simulink model "Quadrature"  (R2024b)
settings: Solver=FixedStepAuto  StartTime=0.0  StopTime=inf  FixedStep=0.1  RelTol=1e-3  EnableMultiTasking=on
libraries: stm32f4xxblockslib x5, stm32g4xxblockslib x3
settings Model: STM32="{\"EncoderBlockForG4\":[{\"ID\":\"Quadrature:1\"},{\"ID\":\"Quadrature:14\"},{\"ID\":\"Quadrature:22\"}],\"DigitalPortRead\":[{\"ID\":\"Quadrature:4\"},{\"ID\":\"Quadrature:10\"},{\"ID\":\"Quadrature:18\"},{\"ID\":\"Quadrature:26\"},{\"ID\":\"Quadrature:27\"}]}"  Creator=spwkp  LastModifiedBy=spwkp
settings OptimizationCC: DefaultParameterBehavior=Inlined  EnhancedBackFolding=on  PassReuseOutputArgsAs=Individual arguments  ZeroExternalMemoryAtStartup=off  ZeroInternalMemoryAtStartup=off  MaxStackSize=512  OptimizeBlockOrder=speed  DifferentSizesBufferReuse=on  OptimizationCustomize=off  EfficientTunableParamExpr=on
settings DebuggingCC: ParameterTunabilityLossMsg=error
settings HardwareCC: ProdBitPerPointer=32  ProdBitPerSizeT=32  ProdBitPerPtrDiffT=32  ProdLargestAtomicInteger=Long  ProdLargestAtomicFloat=Double  ProdWordSize=32  ProdLongLongMode=on  ProdHWDeviceType=ARM Compatible->ARM Cortex-M
settings SFSimCC: MATLABDynamicMemAlloc=off
settings RTWCC: Description=Embedded Coder  SystemTargetFile=ert.tlc  HardwareBoard=STM32G4xx Based  TemplateMakefile=ert_default_tmf  Toolchain=GNU Tools for ARM Embedded Processors
settings CodeAppCC: ForceParamTrailComments=on  IgnoreCustomStorageClasses=off  OperatorAnnotations=on  SimulinkDataObjDesc=on  SFDataObjDesc=on  InsertBlockDesc=on
settings ERTTargetCC: TargetLangStandard=C99 (ISO)  CodeReplacementLibrary=ARM Cortex-M  ExtModeTransport=3  ExtModeStaticAlloc=on  ExtModeStaticAllocSize=2048  ExtModeMexFile=ext_xcp  ExtModeIntrfLevel=Level2 - Open

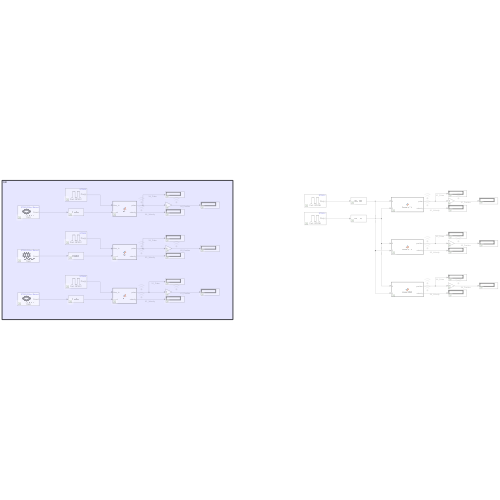
[thumbnail: Simulink's stored preview of the top-level diagram]
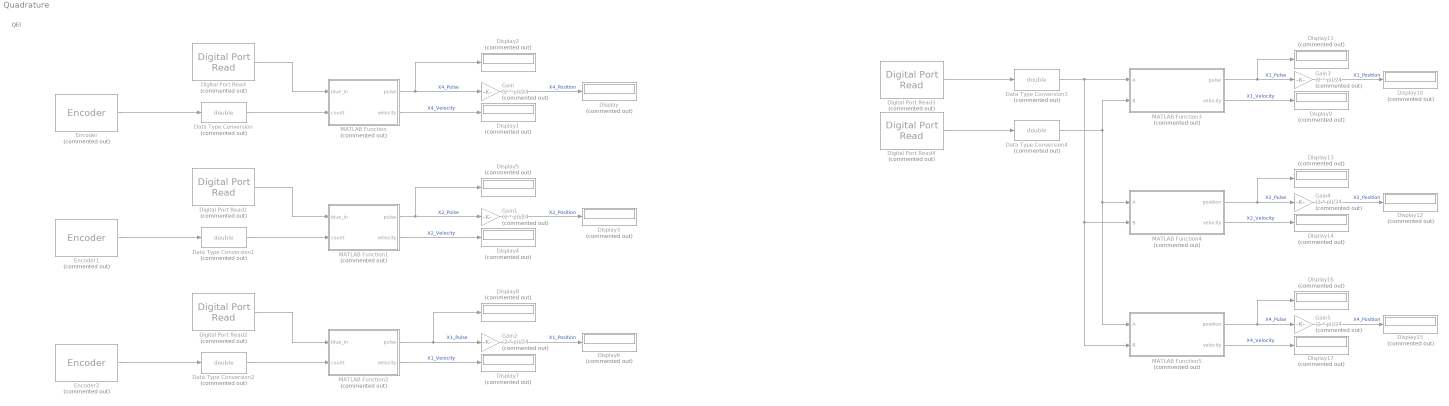
== system Quadrature ==
  note: QEI
  Data Type Conversion{,1..4} (5 alike) : DataTypeConversion  Commented=on  OutDataTypeStr=double  SaturateOnIntegerOverflow=off  RndMeth=Floor
  Digital Port Read : stm32f4xxblockslib/Digital Port Read  Commented=on  PortName=GPIOC  PinNumber=[13]  ReadOperation=on  IOAsArray=on  SampleTime=-1  EnableSimPort=off  hoistedMaskSrc=ECSoC/ECSimCodegen/Digital Port Read
      settings: LibrarySourceBlock=stm32g4xxblockslib/Digital Port Read
  Digital Port Read1 : stm32f4xxblockslib/Digital Port Read  Commented=on  PortName=GPIOC  PinNumber=[13]  ReadOperation=on  IOAsArray=on  SampleTime=-1  EnableSimPort=off  hoistedMaskSrc=ECSoC/ECSimCodegen/Digital Port Read
      settings: LibrarySourceBlock=stm32g4xxblockslib/Digital Port Read
  Digital Port Read2 : stm32f4xxblockslib/Digital Port Read  Commented=on  PortName=GPIOC  PinNumber=[13]  ReadOperation=on  IOAsArray=on  SampleTime=-1  EnableSimPort=off  hoistedMaskSrc=ECSoC/ECSimCodegen/Digital Port Read
      settings: LibrarySourceBlock=stm32g4xxblockslib/Digital Port Read
  Digital Port Read3 : stm32f4xxblockslib/Digital Port Read  Commented=on  PortName=GPIOB  PinNumber=[13]  ReadOperation=on  IOAsArray=on  SampleTime=-1  EnableSimPort=off  hoistedMaskSrc=ECSoC/ECSimCodegen/Digital Port Read
      settings: LibrarySourceBlock=stm32g4xxblockslib/Digital Port Read
  Digital Port Read4 : stm32f4xxblockslib/Digital Port Read  Commented=on  PortName=GPIOB  PinNumber=[14]  ReadOperation=on  IOAsArray=on  SampleTime=-1  EnableSimPort=off  hoistedMaskSrc=ECSoC/ECSimCodegen/Digital Port Read
      settings: LibrarySourceBlock=stm32g4xxblockslib/Digital Port Read
  Display{,1..17} (18 alike) : Display  Commented=on
  Encoder : stm32g4xxblockslib/Encoder  Commented=on  TimerModule=TIM3  EnableResetInput=off  OutputCountAfterFirstIndex=off  OutputValidIndex=off  OutputDirection=off  OutputStatus=off  SampleTime=-1
  Encoder1 : stm32g4xxblockslib/Encoder  Commented=on  TimerModule=TIM4  EnableResetInput=off  OutputCountAfterFirstIndex=off  OutputValidIndex=off  OutputDirection=off  OutputStatus=off  SampleTime=-1
  Encoder2 : stm32g4xxblockslib/Encoder  Commented=on  TimerModule=TIM8  EnableResetInput=off  OutputCountAfterFirstIndex=off  OutputValidIndex=off  OutputDirection=off  OutputStatus=off  SampleTime=-1
  Gain{,1..5} (6 alike) : Gain  Commented=on  Gain=(2 * pi)/24
  MATLAB Function : MATLAB Function  Commented=on  TreatAsAtomicUnit=on
  MATLAB Function1 : MATLAB Function  Commented=on  TreatAsAtomicUnit=on
  MATLAB Function2 : MATLAB Function  Commented=on  TreatAsAtomicUnit=on
  MATLAB Function3 : MATLAB Function  Commented=on  TreatAsAtomicUnit=on
  MATLAB Function4 : MATLAB Function  Commented=on  TreatAsAtomicUnit=on
  MATLAB Function5 : MATLAB Function  Commented=on  TreatAsAtomicUnit=on
  wires:
  Encoder/1 -> Data Type Conversion/1
  Data Type Conversion/1 -> MATLAB Function/2(count)
  Digital Port Read/1 -> MATLAB Function/1(blue_in)
  MATLAB Function/1(pulse) -> Display2/1, Gain/1  "X4_Pulse"
  Gain/1 -> Display/1  "X4_Position"
  MATLAB Function/2(velocity) -> Display1/1  "X4_Velocity"
  MATLAB Function1/1(pulse) -> Display5/1, Gain1/1  "X2_Pulse"
  Encoder1/1 -> Data Type Conversion1/1
  Digital Port Read1/1 -> MATLAB Function1/1(blue_in)
  MATLAB Function1/2(velocity) -> Display4/1  "X2_Velocity"
  Data Type Conversion1/1 -> MATLAB Function1/2(count)
  Gain1/1 -> Display3/1  "X2_Position"
  MATLAB Function2/1(pulse) -> Display8/1, Gain2/1  "X1_Pulse"
  Encoder2/1 -> Data Type Conversion2/1
  Data Type Conversion2/1 -> MATLAB Function2/2(count)
  Gain2/1 -> Display6/1  "X1_Position"
  Digital Port Read2/1 -> MATLAB Function2/1(blue_in)
  MATLAB Function2/2(velocity) -> Display7/1  "X1_Velocity"
  Digital Port Read4/1 -> Data Type Conversion4/1
  Digital Port Read3/1 -> Data Type Conversion3/1
  Data Type Conversion4/1 -> MATLAB Function3/2(B), MATLAB Function5/1(A), MATLAB Function4/1(A)
  MATLAB Function3/2(velocity) -> Display9/1  "X1_Velocity"
  MATLAB Function3/1(pulse) -> Display11/1, Gain3/1  "X1_Pulse"
  Gain3/1 -> Display10/1  "X1_Position"
  Data Type Conversion3/1 -> MATLAB Function5/2(B), MATLAB Function4/2(B), MATLAB Function3/1(A)
  MATLAB Function4/1(position) -> Display13/1, Gain4/1  "X2_Pulse"
  Gain4/1 -> Display12/1  "X2_Position"
  MATLAB Function4/2(velocity) -> Display14/1  "X2_Velocity"
  Gain5/1 -> Display15/1  "X4_Position"
  MATLAB Function5/1(position) -> Display16/1, Gain5/1  "X4_Pulse"
  MATLAB Function5/2(velocity) -> Display17/1  "X4_Velocity"

== matlab function Quadrature/MATLAB Function1 ==
  data: blue_in input; pulse output; count input; velocity output
function [pulse, velocity] = X2(blue_in, count)
    %#codegen
    
    % ประกาศตัวแปร persistent เพื่อเก็บค่าตัวนับก่อนหน้าและตำแหน่งที่คลายห่อก่อนหน้า
    persistent previousCount unwrappedPositionPrev;
    
    % กำหนดค่าเริ่มต้นให้ตัวแปร persistent เมื่อเรียกใช้งานครั้งแรก
    if isempty(previousCount)
        previousCount = count;
        unwrappedPositionPrev = 0;  % กำหนดตำแหน่งคลายห่อเริ่มต้นเป็นศูนย์
    end

    % กำหนดขอบเขตของ encoder
    encoderMax = 65520;   % ค่าสูงสุดสำหรับ encoder แบบ 16-bit (0-65535)
    threshold = encoderMax / 2;  % ค่า threshold สำหรับตรวจจับ overflow หรือ underflow

    % คำนวณค่าความแตกต่างระหว่างค่าปัจจุบันกับค่าก่อนหน้า
    diff_count = count - previousCount;

    % คำนวณความเร็วเชิงมุม (Angular Velocity)
    Ts = 0.01; % กำหนด Sampling Time (เช่น 10ms)
    PPR = 24; % จำนวนพัลส์ต่อรอบ
    velocity = ((diff_count / PPR) / Ts) * 60; % Velocity เป็น RPM

    % ตรวจจับการ overflow และ underflow
    if diff_count > threshold
        % พบการ overflow (เช่น count เปลี่ยนจาก 65535 กลับไปที่ 0)
        pulse = unwrappedPositionPrev + (diff_count - encoderMax);
    elseif diff_count < -threshold
        % พบการ underflow (เช่น count เปลี่ยนจาก 0 เป็น 65535)
        pulse = unwrappedPositionPrev + (diff_count + encoderMax);
    else
        % กรณีปกติที่ไม่มี overflow/underflow
        pulse = unwrappedPositionPrev + diff_count;
    end

    if blue_in == 1
        pulse = 0;
        velocity = 0;
    end
    % อัปเดตตัวแปร persistent เพื่อใช้ในรอบถัดไป
    previousCount = count;
    unwrappedPositionPrev = pulse; 
end

== matlab function Quadrature/MATLAB Function ==
  data: blue_in input; pulse output; count input; velocity output
function [pulse, velocity] = X4(blue_in, count)
    %#codegen
    
    % ประกาศตัวแปร persistent เพื่อเก็บค่าตัวนับก่อนหน้าและตำแหน่งที่คลายห่อก่อนหน้า
    persistent previousCount unwrappedPositionPrev;
    
    % กำหนดค่าเริ่มต้นให้ตัวแปร persistent เมื่อเรียกใช้งานครั้งแรก
    if isempty(previousCount)
        previousCount = count;
        unwrappedPositionPrev = 0;  % กำหนดตำแหน่งคลายห่อเริ่มต้นเป็นศูนย์
    end

    % กำหนดขอบเขตของ encoder
    encoderMax = 65520;   % ค่าสูงสุดสำหรับ encoder แบบ 16-bit (0-65535)
    threshold = encoderMax / 2;  % ค่า threshold สำหรับตรวจจับ overflow หรือ underflow

    % คำนวณค่าความแตกต่างระหว่างค่าปัจจุบันกับค่าก่อนหน้า
    diff_count = count - previousCount;

    % คำนวณความเร็วเชิงมุม (Angular Velocity)
    Ts = 0.01; % กำหนด Sampling Time (เช่น 10ms)
    PPR = 24; % จำนวนพัลส์ต่อรอบ
    velocity = ((diff_count / PPR) / Ts) * 60; % Velocity เป็น RPM

    % ตรวจจับการ overflow และ underflow
    if diff_count > threshold
        % พบการ overflow (เช่น count เปลี่ยนจาก 65535 กลับไปที่ 0)
        pulse = unwrappedPositionPrev + (diff_count - encoderMax);
    elseif diff_count < -threshold
        % พบการ underflow (เช่น count เปลี่ยนจาก 0 เป็น 65535)
        pulse = unwrappedPositionPrev + (diff_count + encoderMax);
    else
        % กรณีปกติที่ไม่มี overflow/underflow
        pulse = unwrappedPositionPrev + diff_count;
    end

    if blue_in == 1
        pulse = 0;
        velocity = 0;
    end
    % อัปเดตตัวแปร persistent เพื่อใช้ในรอบถัดไป
    previousCount = count;
    unwrappedPositionPrev = pulse; 
end

== matlab function Quadrature/MATLAB Function2 ==
  data: blue_in input; pulse output; count input; velocity output
function [pulse, velocity] = X1(blue_in, count)
    %#codegen
    
    % ประกาศตัวแปร persistent เพื่อเก็บค่าตัวนับก่อนหน้าและตำแหน่งที่คลายห่อก่อนหน้า
    persistent previousCount unwrappedPositionPrev;
    
    % กำหนดค่าเริ่มต้นให้ตัวแปร persistent เมื่อเรียกใช้งานครั้งแรก
    if isempty(previousCount)
        previousCount = count;
        unwrappedPositionPrev = 0;  % กำหนดตำแหน่งคลายห่อเริ่มต้นเป็นศูนย์
    end

    % กำหนดขอบเขตของ encoder
    encoderMax = 65520;   % ค่าสูงสุดสำหรับ encoder แบบ 16-bit (0-65535)
    threshold = encoderMax / 2;  % ค่า threshold สำหรับตรวจจับ overflow หรือ underflow

    % คำนวณค่าความแตกต่างระหว่างค่าปัจจุบันกับค่าก่อนหน้า
    diff_count = count - previousCount;

    % คำนวณความเร็วเชิงมุม (Angular Velocity)
    Ts = 0.01; % กำหนด Sampling Time (เช่น 10ms)
    PPR = 24; % จำนวนพัลส์ต่อรอบ
    velocity = ((diff_count / PPR) / Ts) * 60; % Velocity เป็น RPM

    % ตรวจจับการ overflow และ underflow
    if diff_count > threshold
        % พบการ overflow (เช่น count เปลี่ยนจาก 65535 กลับไปที่ 0)
        pulse = unwrappedPositionPrev + (diff_count - encoderMax);
    elseif diff_count < -threshold
        % พบการ underflow (เช่น count เปลี่ยนจาก 0 เป็น 65535)
        pulse = unwrappedPositionPrev + (diff_count + encoderMax);
    else
        % กรณีปกติที่ไม่มี overflow/underflow
        pulse = unwrappedPositionPrev + diff_count;
    end

    if blue_in == 1
        pulse = 0;
        velocity = 0;
    end
    % อัปเดตตัวแปร persistent เพื่อใช้ในรอบถัดไป
    previousCount = count;
    unwrappedPositionPrev = pulse; 
end

== matlab function Quadrature/MATLAB Function3 ==
  data: A input double size=[1 1]; pulse output; B input double size=[1 1]; velocity output
function [pulse, velocity] = EncoderX1(A, B)
    % readEncoderX1 - Read encoder position and velocity in RPM using X1 mode with polling
    % A and B are the input signals from the encoder channels A and B
    % position returns the current encoder position, counting forward and backward
    % velocity_rpm returns the calculated velocity in RPM based on position change and fixed sample time
   
    persistent lastA count lastCount;
    if isempty(lastA) || isempty(count) || isempty(lastCount)
        % Initialize variables if not set
        lastA = 0;
        count = 0;
        lastCount = 0;
    end
    
    % Read current states of A and B
    currentA = A;  
    currentB = B;  
    
    % Check for rising edge of A (from 0 to 1)
    if lastA ~= currentA
        % Determine direction based on the state of B
        if currentB == 0 && currentA == 1
            count = count + 1;  % Forward count
        elseif currentB == 1 && currentA == 1
            count = count - 1;  % Backward count
        end
    end
    
    % Calculate velocity in counts per 0.01 sec and convert to RPM
    velocity = (count - lastCount) * 6000;  % Scale for RPM based on 0.01s sampling time
    
    % Update last values for the next polling cycle
    lastA = currentA;
    lastCount = count;
    
    % Return the current position count and calculated velocity in RPM
    pulse = count;
end

== matlab function Quadrature/MATLAB Function4 ==
  data: A input double size=[1 1]; position output; B input double size=[1 1]; velocity output
function [position, velocity] = EncoderX2(A, B)
    % EncoderX2 - Read encoder position and velocity in RPM using X2 mode with polling
    % A and B are the input signals from the encoder channels A and B
    % position returns the current encoder position, counting forward and backward
    % velocity returns the calculated velocity in RPM based on position change and fixed sample time
    
    persistent lastA lastB count lastCount;
    
    % Initialize variables if not set
    if isempty(lastA)
        lastA = 0;
        lastB = 0;
        count = 0;
        lastCount = 0;
    end
    
    % Read current states of A and B
    currentA = A;  
    currentB = B;  
    
    % Check for rising edge of A
    if lastA ~= currentA && currentA == 1
        % Determine direction based on the state of B
        if currentB == 0
            count = count + 1;  % Forward count
        else
            count = count - 1;  % Backward count
        end
    end
    
    % Check for falling edge of A
    if lastA ~= currentA && currentA == 0
        % Determine direction based on the state of B
        if currentB == 0
            count = count - 1;  % Backward count
        else
            count = count + 1;  % Forward count
        end
    end
    
    % Calculate velocity in counts per 0.01 sec and convert to RPM
    velocity = (count - lastCount) * 6000;  % Scale for RPM based on 0.01s sampling time
    
    % Update last values for the next polling cycle
    lastA = currentA;
    lastB = currentB;
    lastCount = count;
    
    % Return the current position count and calculated velocity in RPM
    position = count;
end

== matlab function Quadrature/MATLAB Function5 ==
  data: A input double size=[1 1]; position output; B input double size=[1 1]; velocity output
function [position, velocity] = EncoderX2(A, B)
    % EncoderX2 - Read encoder position and velocity in RPM using X2 mode with polling
    % A and B are the input signals from the encoder channels A and B
    % position returns the current encoder position, counting forward and backward
    % velocity returns the calculated velocity in RPM based on position change and fixed sample time
    
    persistent lastA lastB count lastCount;
    
    % Initialize variables if not set
    if isempty(lastA)
        lastA = 0;
        lastB = 0;
        count = 0;
        lastCount = 0;
    end
    
    % Read current states of A and B
    currentA = A;  
    currentB = B;  
    
    % Check for rising edge of A
    if lastA ~= currentA && currentA == 1
        % Determine direction based on the state of B
        if currentB == 0
            count = count + 1;  % Forward count
        else
            count = count - 1;  % Backward count
        end
    end
    
    % Check for falling edge of A
    if lastA ~= currentA && currentA == 0
        % Determine direction based on the state of B
        if currentB == 0
            count = count - 1;  % Backward count
        else
            count = count + 1;  % Forward count
        end
    end

    % Check for rising edge of B
    if lastB ~= currentB && currentB == 1
        % Determine direction based on the state of B
        if currentA == 0
            count = count + 1;  % Forward count
        else
            count = count - 1;  % Backward count
        end
    end

    % Check for falling edge of B
    if lastB ~= currentB && currentB == 0
        % Determine direction based on the state of B
        if currentB == 0
            count = count - 1;  % Backward count
        else
            count = count + 1;  % Forward count
        end
    end

    % Calculate velocity in counts per 0.01 sec and convert to RPM
    velocity = (count - lastCount) * 6000;  % Scale for RPM based on 0.01s sampling time
    
    % Update last values for the next polling cycle
    lastA = currentA;
    lastB = currentB;
    lastCount = count;
    
    % Return the current position count and calculated velocity in RPM
    position = count;
end
